simulink model "metro"  (R2016a)
settings: Solver=VariableStepAuto  StartTime=0.0  StopTime=100000  RelTol=1e-3
settings Model: Creator=ferson  LastModifiedBy=ferson

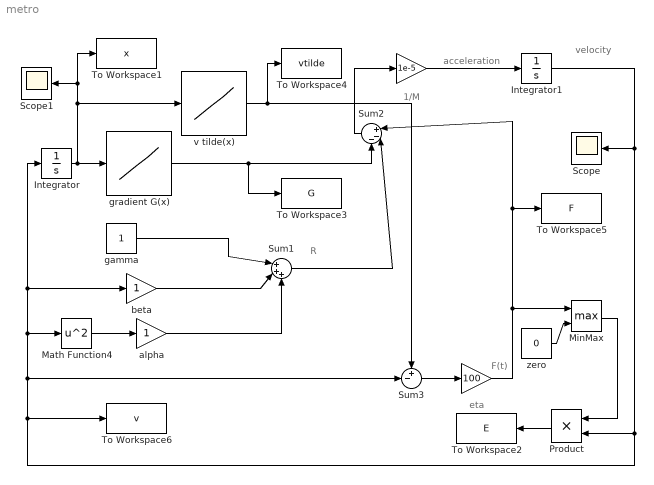
== system metro ==
  note: eta
  note: 1/M
  note: velocity
  note: acceleration
  note: F(t)
  note: R
  " " : Gain  Gain=100
  "  " : Gain  Gain=1e-5
  Integrator : Integrator
  Integrator1 : Integrator
  Math Function4 : Math  Operator=square  SaturateOnIntegerOverflow=on
  MinMax : MinMax  Function=max  Inputs=2
  "Product " : Product  Inputs=**
  Scope : Scope
  Scope1 : Scope
  Sum1 : Sum  Inputs=|+++
  Sum2 : Sum  Inputs=|+--
  Sum3 : Sum  Inputs=+-|
  To Workspace1 : ToWorkspace  VariableName=x  SaveFormat=Timeseries  SampleTime=-1
  To Workspace2 : ToWorkspace  VariableName=E  SaveFormat=Timeseries  SampleTime=-1
  To Workspace3 : ToWorkspace  VariableName=G  SaveFormat=Timeseries  SampleTime=-1
  To Workspace4 : ToWorkspace  VariableName=vtilde  SaveFormat=Timeseries  SampleTime=-1
  To Workspace5 : ToWorkspace  VariableName=F  SaveFormat=Timeseries  SampleTime=-1
  To Workspace6 : ToWorkspace  VariableName=v  SaveFormat=Timeseries  SampleTime=-1
  alpha : Gain
  beta : Gain
  gamma : Constant
  gradient G(x) : Lookup_n-D  NumberOfTableDimensions=1  BreakpointsForDimension1=[-5:5]  Table=0.1 * tanh([-5:5])  InternalRulePriority=Speed  RndMeth=Simplest  InputSameDT=on
  v tilde(x) : Lookup_n-D  NumberOfTableDimensions=1  BreakpointsForDimension1=[-5:5]  Table=2-0.1*tanh([-5:5])  InternalRulePriority=Speed  RndMeth=Simplest  InputSameDT=on
  zero : Constant  Value=0
  wires:
  Integrator1/1 -> Integrator/1, beta/1, Math Function4/1, Sum3/2, To Workspace6/1, "Product "/2, Scope/1
  alpha/1 -> Sum1/3
  gamma/1 -> Sum1/1
  Math Function4/1 -> alpha/1
  beta/1 -> Sum1/2
  Sum1/1 -> Sum2/2
  Integrator/1 -> Scope1/1, To Workspace1/1, v tilde(x)/1, gradient G(x)/1
  gradient G(x)/1 -> To Workspace3/1, Sum2/3
  Sum3/1 -> " "/1
  " "/1 -> MinMax/1, To Workspace5/1, Sum2/1
  Sum2/1 -> "  "/1
  "  "/1 -> Integrator1/1
  zero/1 -> MinMax/2
  MinMax/1 -> "Product "/1
  "Product "/1 -> To Workspace2/1
  v tilde(x)/1 -> To Workspace4/1, Sum3/1
